simulink model "incubator_data"  (R2023a)
settings: Solver=VariableStepAuto  StartTime=0.0  StopTime=10000  RelTol=1e-3
values from neighbouring files (symbols this model uses):
  Acv = 0.9 * Sa    (= 0.163689221901)    [incubator.m]
  Anet = Amat - As    (= 0.1872)    [incubator.m]
  Ar = 0.555 * Sa    (= 0.100941686839)    [incubator.m]
  As = 0.36*0.15    (= 0.054)    [incubator.m]
  Awi = 1.2    [incubator.m]
  bf = 0.18*60 / 1000    (= 0.0108)    [incubator.m]
  cp_b = 3770    [incubator.m]
  cp_co = 3470    [incubator.m]
  cpa = 1005    [incubator.m]
  cpa_skin = 3400    [incubator.m]
  cpm = 1500    [incubator.m]
  cpw = 4e7    (= 40000000)    [incubator.m]
  eps_s = 0.97    [incubator.m]
  epsilon_w = 0.9    [incubator.m]
  Evap = 0.15e-9    (= 1.5e-10)    [incubator.m]
  hf_g = 2.343e6    (= 2343000)    [incubator.m]
  hfg = 2.257e6    (= 2257000)    [incubator.m]
  hien = hscv    (= 0.464725290588)    [incubator.m]
  hscv = (Nu * Ka) / Dsph    (= 0.464725290588)    [incubator.m]
  IV = 3.3e-6    (= 3.3e-06)    [incubator.m]
  K_c = 0.6    [incubator.m]
  Kmat = 0.07    [incubator.m]
  kplex = 0.189    [incubator.m]
  m = 2.46    [incubator.m]
  ma = 0.02    [incubator.m]
  mco = m_co    (= 1.41420774897)    [incubator.m]
  ms = th_s * rho_s * Sa    (= 1.04579225103)    [incubator.m]
  mw = rho_w * th_w * Awi    (= 12.72)    [incubator.m]
  Qmet = mrst*Sa    (= 5.94999408995)    [incubator.m]
  rho_a = 1.2    [incubator.m]
  rho_bl = 1060    [incubator.m]
  rho_c = 1050    [incubator.m]
  rho_w = 1060    [incubator.m]
  Sa = m^0.75/10.8    (= 0.181876913223)    [incubator.m]
  sigma = 5.670e-8    (= 5.67e-08)    [incubator.m]
  th_w = 0.01    [incubator.m]
  thm = 0.04    [incubator.m]
  Wa = 0.010    (= 0.01)    [incubator.m]
  Wex = 44e-6/1.184e-3    (= 0.0371621621622)    [incubator.m]
settings Model: Creator=ACER  LastModifiedBy=ACER

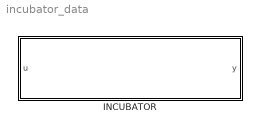
== system incubator_data ==
  INCUBATOR : Subsystem

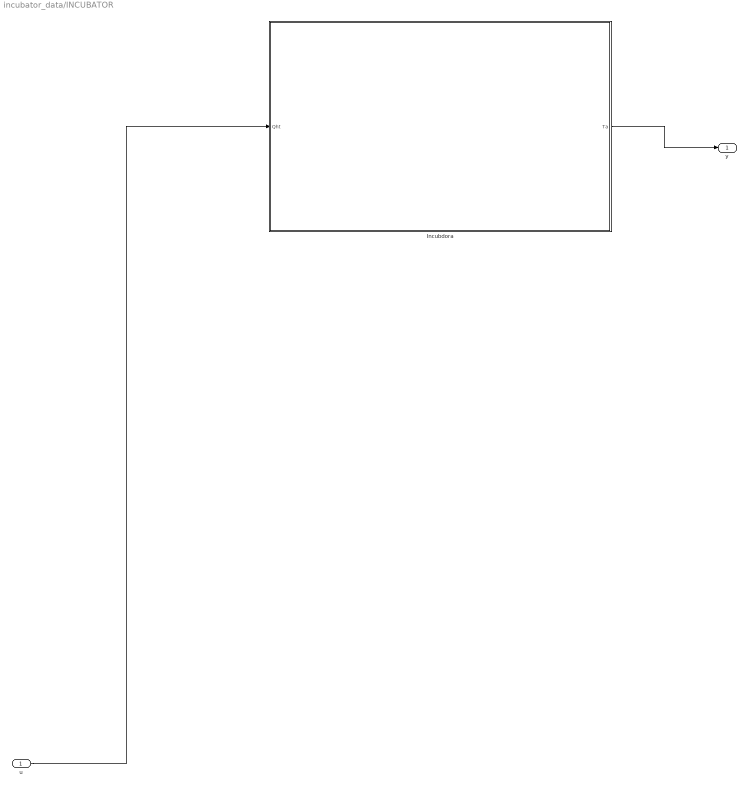
== system incubator_data/INCUBATOR ==
  u : Inport
  Incubdora : Subsystem
  y : Outport
  wires:
  u/1 -> Incubdora/1(Qht)
  Incubdora/1(Ta) -> y/1

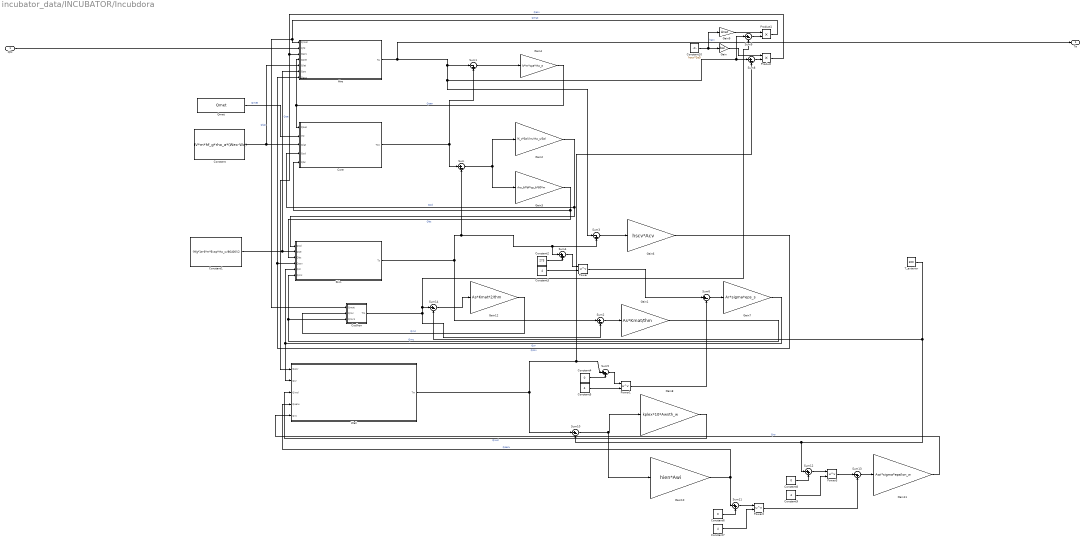
== system incubator_data/INCUBATOR/Incubdora ==
  Qht : Inport
  Aire : Subsystem
  Coclhon : Subsystem
  Constant : Constant  Value=IV*m*hf_g*rho_a*(Wex-Wa)
  Constant1 : Constant  Value=(hfg*1e-6*m*Evap*rho_w/86400)/2
  Constant10 : Constant  Value=hscv*1e5
  Constant2 : Constant  Value=273
  Constant{3,5,7,9} (4 alike) : Constant  Value=4
  Constant4 : Constant  Value=0
  Constant6 : Constant  Value=0
  Constant8 : Constant  Value=0
  Core : Subsystem
  Gain : Gain  Gain=Awi
  Gain1 : Gain  Gain=As*Kmat/thm
  Gain10 : Gain  Gain=hien*Awi
  Gain11 : Gain  Gain=Awi*sigma*epsilon_w
  Gain12 : Gain  Gain=As*Kmat*2/thm
  Gain2 : Gain  Gain=(K_c*Sa)/(m/rho_c/Sa)
  Gain3 : Gain  Gain=rho_bl*bf*cp_b*80*m
  Gain4 : Gain  Gain=IV*m*cpa*rho_a
  Gain6 : Gain  Gain=hscv*Acv
  Gain7 : Gain  Gain=Ar*sigma*eps_s
  Gain8 : Gain  Gain=kplex*10*Awi/th_w
  Gain9 : Gain  Gain=Anet
  Power{,1..3} (4 alike) : Math  Operator=pow
  Product : Product
  Product1 : Product
  Qmet : Constant  Value=Qmet
  Skin : Subsystem
  Sum{,2,6,8..10,14} (7 alike) : Sum  Inputs=|+-
  Sum1 : Sum  Inputs=|-+
  Sum{4..5,11..12} (4 alike) : Sum  Inputs=|++
  Sum13 : Sum  Inputs=|-+
  Sum3 : Sum  Inputs=|-+
  T_exterior : Constant  Value=300
  Wall : Subsystem
  Ta : Outport
  wires:
  Product1/1 -> Coclhon/1(Qmat), Aire/1(Qmat)  "Qmat"
  Gain8/1 -> Wall/3(Qiwd)  "Qiwd"
  Product/1 -> Wall/1(Qacv), Aire/3(Qacv)  "Qacv"
  Power/1 -> Sum6/1
  Gain2/1 -> Skin/1(Qcd), Core/4(Qcd)  "Qcd"
  Sum1/1 -> Gain4/1
  Constant3/1 -> Power/2
  Aire/1(Ta) -> Ta/1, Sum9/1, Sum8/1, Sum3/1, Sum1/1
  Qmet/1 -> Core/2(In2)  "Qmet"
  Power1/1 -> Sum6/2
  Sum4/1 -> Power/1
  Sum3/1 -> Gain6/1
  Sum14/1 -> Gain12/1
  Coclhon/1(Tm) -> Sum2/2, Sum14/1, Sum9/2
  Sum5/1 -> Power1/1
  Constant2/1 -> Sum4/2
  Gain7/1 -> Wall/2(Qsr), Skin/5(Qsr)  "Qsr"
  Gain4/1 -> Aire/4(Qsen), Core/1(Qsen)  "Qsen"
  Constant1/1 -> Aire/6(Qse), Skin/2(Qse)  "Qse"
  Sum/1 -> Gain3/1, Gain2/1
  Gain11/1 -> Wall/5(Qro)  "Qro"
  Sum13/1 -> Gain11/1
  Constant8/1 -> Sum12/2
  Gain9/1 -> Product1/1
  Gain1/1 -> Skin/6(Qmc), Coclhon/3(Qmc1)  "Qmc"
  Core/1(Tco) -> Sum1/2, Sum/1
  Constant4/1 -> Sum5/2
  Wall/1(Tw) -> Sum8/2, Sum5/1, Sum10/1
  Skin/1(Ts) -> Sum4/1, Sum3/2, Sum/2, Sum2/1
  Constant5/1 -> Power1/2
  Constant6/1 -> Sum11/2
  Sum2/1 -> Gain1/1
  Gain/1 -> Product/1
  Constant10/1 -> Gain9/1, Gain/1  "hacv"
  Gain6/1 -> Aire/7(Qscv), Skin/4(Qscv)  "Qscv"
  Gain3/1 -> Skin/3(Qbc), Core/5(Qbc)  "Qbc"
  Sum8/1 -> Product/2
  Gain10/1 -> Wall/4(Qoenv), Sum11/1  "Qoenv"
  Power2/1 -> Sum13/2
  T_exterior/1 -> Sum14/2, Sum12/1, Sum10/2
  Sum12/1 -> Power3/1
  Gain12/1 -> Coclhon/2(Qmc)  "Qmc"
  Sum10/1 -> Gain10/1, Gain8/1
  Constant7/1 -> Power2/2
  Constant9/1 -> Power3/2
  Sum6/1 -> Gain7/1
  Sum9/1 -> Product1/2
  Sum11/1 -> Power2/1
  Power3/1 -> Sum13/1
  Constant/1 -> Aire/5(Qlat), Core/3(Qlat)  "Qlat"
  Qht/1 -> Aire/2(Qht)

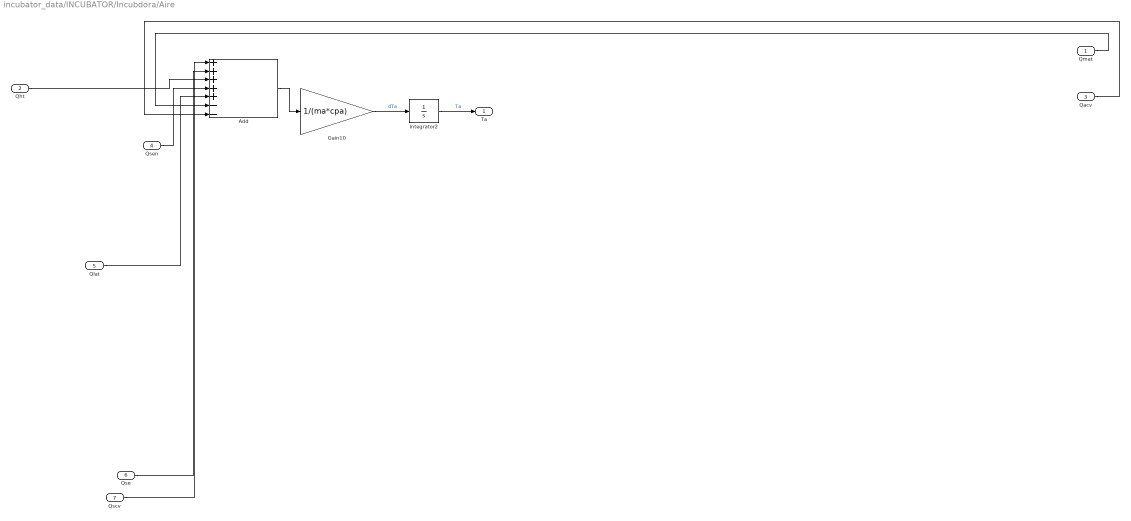
== system incubator_data/INCUBATOR/Incubdora/Aire ==
  Qmat : Inport
  Qht : Inport  Port=2
  Qacv : Inport  Port=3
  Qsen : Inport  Port=4
  Qlat : Inport  Port=5
  Qse : Inport  Port=6
  Qscv : Inport  Port=7
  Add : Sum  Inputs=+++++--
  Gain10 : Gain  Gain=1/(ma*cpa)
  Integrator2 : Integrator  InitialCondition=300
  Ta : Outport
  wires:
  Qse/1 -> Add/2
  Qsen/1 -> Add/4
  Qlat/1 -> Add/5
  Add/1 -> Gain10/1
  Integrator2/1 -> Ta/1  "Ta"
  Gain10/1 -> Integrator2/1  "dTa"
  Qht/1 -> Add/3
  Qscv/1 -> Add/1
  Qacv/1 -> Add/7
  Qmat/1 -> Add/6

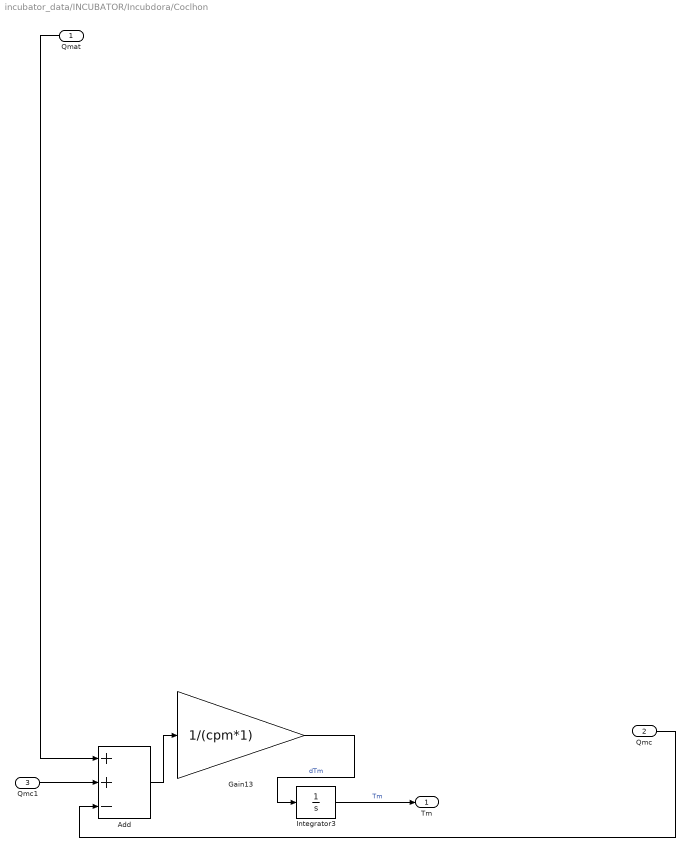
== system incubator_data/INCUBATOR/Incubdora/Coclhon ==
  Qmat : Inport
  Qmc : Inport  Port=2
  Qmc1 : Inport  Port=3
  Add : Sum  Inputs=++-
  Gain13 : Gain  Gain=1/(cpm*1)
  Integrator3 : Integrator  InitialCondition=308
  Tm : Outport
  wires:
  Integrator3/1 -> Tm/1  "Tm"
  Add/1 -> Gain13/1
  Gain13/1 -> Integrator3/1  "dTm"
  Qmc/1 -> Add/3
  Qmat/1 -> Add/1
  Qmc1/1 -> Add/2

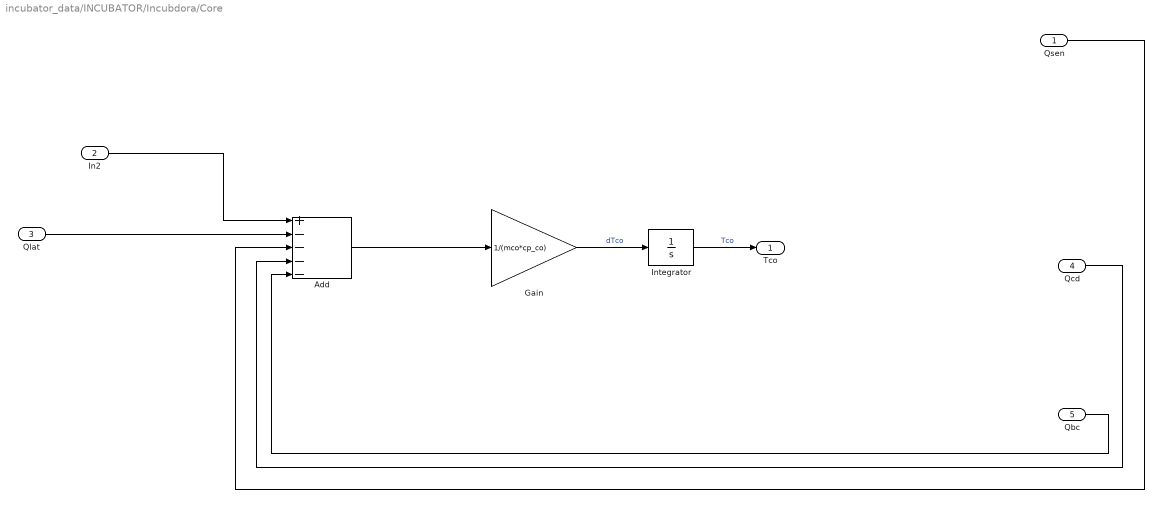
== system incubator_data/INCUBATOR/Incubdora/Core ==
  Qsen : Inport
  In2 : Inport  Port=2
  Qlat : Inport  Port=3
  Qcd : Inport  Port=4
  Qbc : Inport  Port=5
  Add : Sum  Inputs=+----
  Gain : Gain  Gain=1/(mco*cp_co)
  Integrator : Integrator  InitialCondition=308
  Tco : Outport
  wires:
  Qlat/1 -> Add/2
  Gain/1 -> Integrator/1  "dTco"
  Qbc/1 -> Add/5
  Qcd/1 -> Add/4
  Integrator/1 -> Tco/1  "Tco"
  Add/1 -> Gain/1
  In2/1 -> Add/1
  Qsen/1 -> Add/3

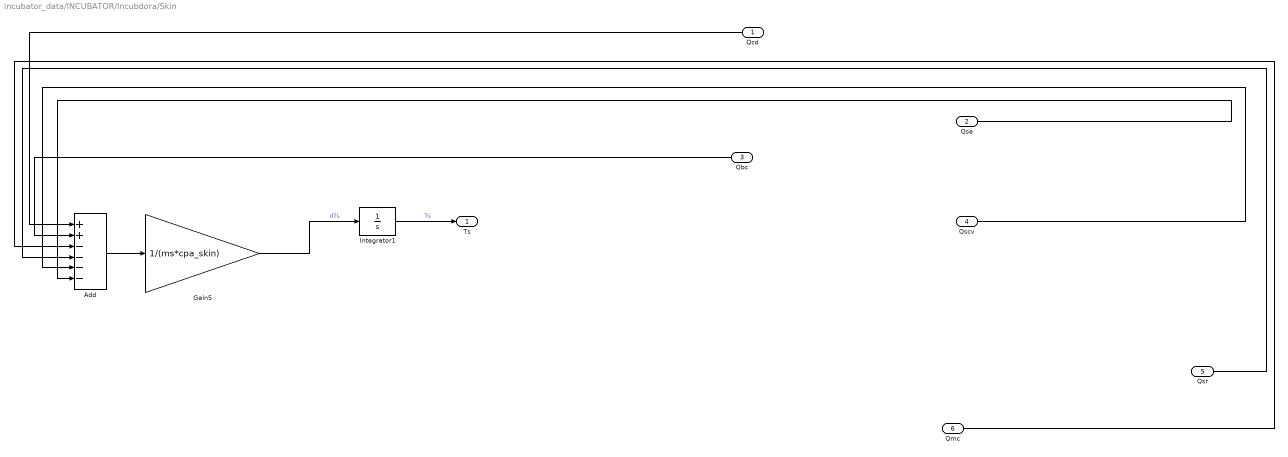
== system incubator_data/INCUBATOR/Incubdora/Skin ==
  Qcd : Inport
  Qse : Inport  Port=2
  Qbc : Inport  Port=3
  Qscv : Inport  Port=4
  Qsr : Inport  Port=5
  Qmc : Inport  Port=6
  Add : Sum  Inputs=++----
  Gain5 : Gain  Gain=1/(ms*cpa_skin)
  Integrator1 : Integrator  InitialCondition=308
  Ts : Outport
  wires:
  Qbc/1 -> Add/2
  Qscv/1 -> Add/5
  Add/1 -> Gain5/1
  Gain5/1 -> Integrator1/1  "dTs"
  Qse/1 -> Add/6
  Qmc/1 -> Add/3
  Qsr/1 -> Add/4
  Integrator1/1 -> Ts/1  "Ts"
  Qcd/1 -> Add/1

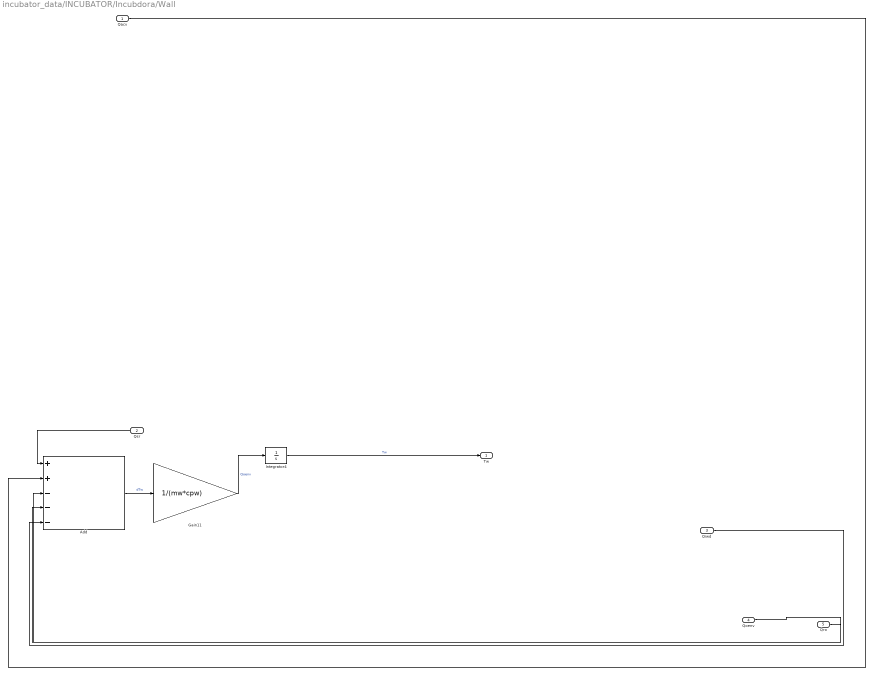
== system incubator_data/INCUBATOR/Incubdora/Wall ==
  Qacv : Inport
  Qsr : Inport  Port=2
  Qiwd : Inport  Port=3
  Qoenv : Inport  Port=4
  Qro : Inport  Port=5
  Add : Sum  Inputs=++---
  Gain11 : Gain  Gain=1/(mw*cpw)
  Integrator4 : Integrator  InitialCondition=308
  Tw : Outport
  wires:
  Add/1 -> Gain11/1  "dTw"
  Qsr/1 -> Add/1
  Qacv/1 -> Add/2
  Gain11/1 -> Integrator4/1  "Qoenv"
  Qoenv/1 -> Add/4
  Qiwd/1 -> Add/5
  Qro/1 -> Add/3
  Integrator4/1 -> Tw/1  "Tw"
